simulink model "battery_charge_and_discharge"  (R2022a)
settings: Solver=ode4  StartTime=0.0  StopTime=Sim_Time  FixedStep=0.001  RelTol=1e-3
values from neighbouring files (symbols this model uses):
  Cn = 2.3 * 3600    (= 8280)    [params_setup.m]
  I = -2.3    [params_setup.m]
  initialCurrent = Cn    (= 8280)    [params_setup.m]
  OCV = Data(:,2)    [read_data.m]
  R_Charge = Data(:,3)    [read_data.m]
  R_Discharge = Data(:,4)    [read_data.m]
  SOC = Data(:,1)    [read_data.m]
settings Model: Creator=stakk  LastModifiedBy=stakk

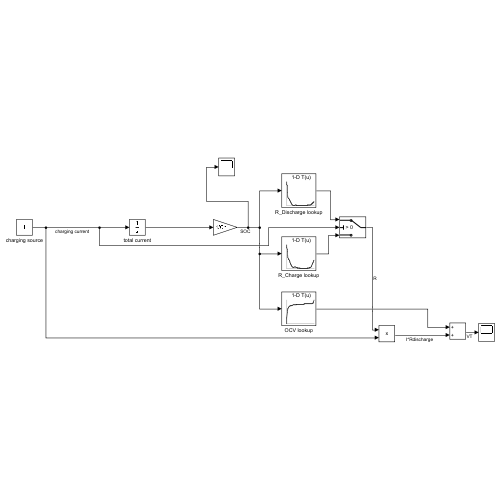
[thumbnail: Simulink's stored preview of the top-level diagram]
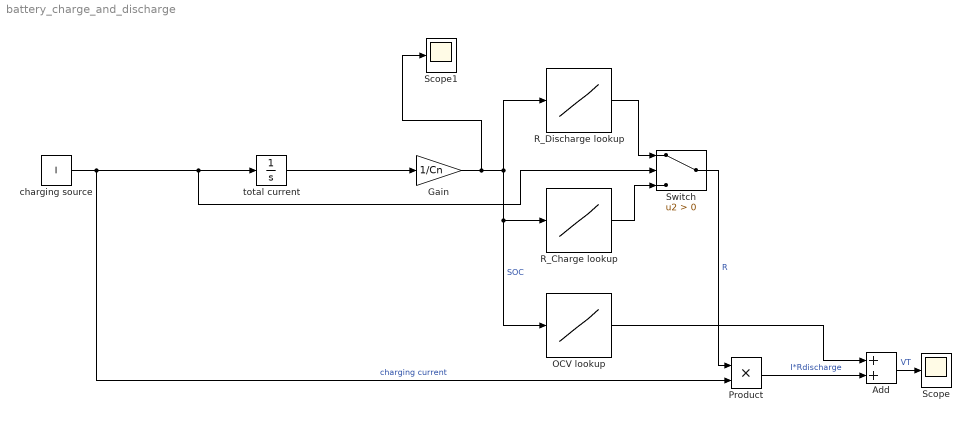
== system battery_charge_and_discharge ==
  Add : Sum
  Gain : Gain  Gain=1/Cn
  OCV lookup : Lookup_n-D  NumberOfTableDimensions=1  BreakpointsForDimension1=SOC  Table=OCV  InternalRulePriority=Speed  RndMeth=Simplest
  Product : Product
  R_Charge lookup : Lookup_n-D  NumberOfTableDimensions=1  BreakpointsForDimension1=SOC  Table=R_Charge  InternalRulePriority=Speed  RndMeth=Simplest
  R_Discharge lookup : Lookup_n-D  NumberOfTableDimensions=1  BreakpointsForDimension1=SOC  Table=R_Discharge  InternalRulePriority=Speed  RndMeth=Simplest
  Scope : Scope
  Scope1 : Scope
  Switch : Switch  Criteria=u2 > Threshold  SaturateOnIntegerOverflow=off  InputSameDT=off
  charging source : Constant  Value=I
  total current : Integrator  InitialCondition=initialCurrent
  wires:
  charging source/1 -> Product/2, Switch/2, total current/1  "charging current"
  total current/1 -> Gain/1
  Switch/1 -> Product/1  "R"
  Product/1 -> Add/2  "I*Rdischarge"
  Add/1 -> Scope/1  "VT"
  Gain/1 -> R_Discharge lookup/1, OCV lookup/1, R_Charge lookup/1, Scope1/1  "SOC"
  R_Charge lookup/1 -> Switch/3
  R_Discharge lookup/1 -> Switch/1
  OCV lookup/1 -> Add/1
